simulink model "fs"  (R2021a)
settings: Solver=FixedStepAuto  StartTime=0.0  StopTime=inf  FixedStep=0.05  RelTol=1e-3
undefined symbols (not defined in the file): Angular, Linear
libraries: robotlib x19, simulink x1
settings Model: Creator=ivory  LastModifiedBy=refulgent
settings SolverCC: AlgebraicLoopSolver=TrustRegion
settings OptimizationCC: EnhancedBackFolding=on  PassReuseOutputArgsAs=Individual arguments  ZeroExternalMemoryAtStartup=off  ZeroInternalMemoryAtStartup=off  MaxStackSize=64  OptimizeBlockOrder=speed  DifferentSizesBufferReuse=on  OptimizationCustomize=off  EfficientTunableParamExpr=on
settings DebuggingCC: ParameterTunabilityLossMsg=error  SFMachineParentedDataDiag=warning
settings HardwareCC: ProdBitPerPointer=32  ProdBitPerSizeT=32  ProdBitPerPtrDiffT=32  ProdLargestAtomicFloat=None  ProdIntDivRoundTo=Undefined  ProdEndianess=Unspecified  ProdWordSize=32  ProdHWDeviceType=Generic->Unspecified (assume 32-bit Generic)
settings SFSimCC: MATLABDynamicMemAlloc=off  SimTargetLang=C++
settings RTWCC: SystemTargetFile=ert.tlc  HardwareBoard=Robot Operating System (ROS)  TLCOptions="-aInlineSetEventsForThisBaseRateFcn=TLC_FALSE -aSuppressMultiTaskScheduler=TLC_FALSE  -aRateBasedStepFcn=0"  TemplateMakefile=ert_default_tmf  GenerateReport=on  Toolchain=Catkin  IncludeHyperlinkInReport=on  LaunchReport=on  TargetLang=C++  GenerateTraceInfo=on  GenerateTraceReport=on  GenerateTraceReportSl=on  GenerateTraceReportSf=on  GenerateTraceReportEml=on
settings CodeAppCC: ForceParamTrailComments=on  IgnoreCustomStorageClasses=off  OperatorAnnotations=on  SimulinkDataObjDesc=on  SFDataObjDesc=on  InsertBlockDesc=on
settings ERTTargetCC: SupportContinuousTime=on  SupportVariableSizeSignals=on

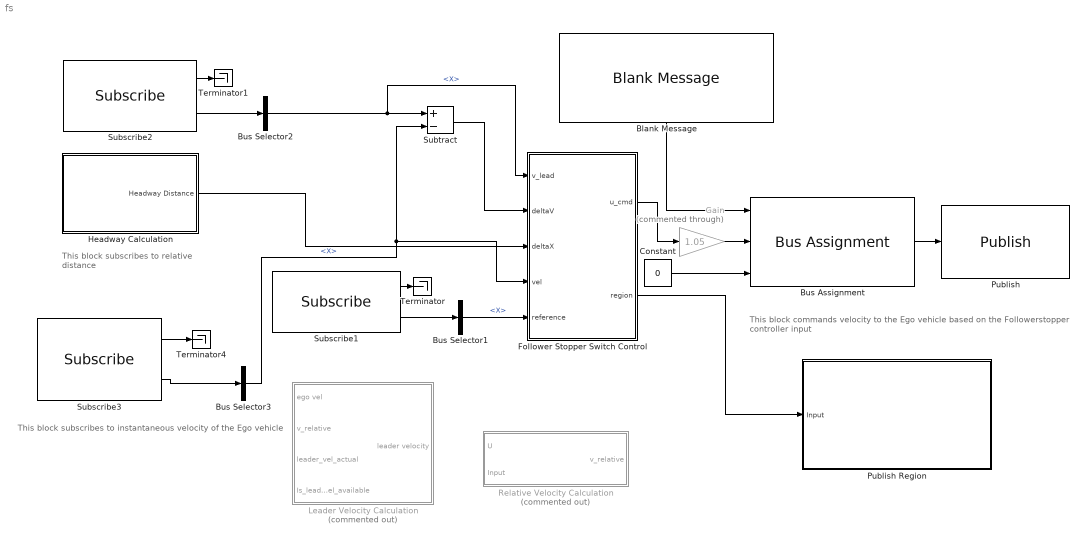
== system fs ==
  note: This block subscribes to
      | instantaneous velocity of the Ego vehicle
  note: This block subscribes
      | to relative distance
  note: This block commands velocity to the Ego vehicle based
      | on the Followerstopper controller input
  Blank Message : robotlib/Blank Message  messageClass=Message  entityType=geometry_msgs/Twist  messageType=geometry_msgs/Twist  SampleTime=inf  legacyBusStruct=off
  Bus Assignment : BusAssignment  AssignedSignals=Linear.X,Angular.Z
  Bus Selector1 : BusSelector  OutputSignals=Linear.X
  Bus Selector2 : BusSelector  OutputSignals=Linear.X
  Bus Selector3 : BusSelector  OutputSignals=Linear.X
  Constant : Constant  Value=0
  Follower Stopper Switch Control : Subsystem
  Gain : Gain  Commented=through  Gain=1.05
  Headway Calculation : Subsystem
  Leader Velocity Calculation : Subsystem  Commented=on
  Publish : robotlib/Publish  topicSource=Specify your own  topic=cmd_vel  messageType=geometry_msgs/Twist  legacyBusStruct=off  messageQueueLength=1
  Publish Region : Subsystem
  Relative Velocity Calculation : Subsystem  Commented=on
  Subscribe1 : robotlib/Subscribe  topicSource=Specify your own  topic=v_ref  messageType=geometry_msgs/Twist  SampleTime=-1  legacyBusStruct=off  messageQueueLength=1
  Subscribe2 : robotlib/Subscribe  topicSource=Specify your own  topic=leader_vel  messageType=geometry_msgs/Twist  SampleTime=-1  legacyBusStruct=off  messageQueueLength=1
  Subscribe3 : robotlib/Subscribe  topicSource=Specify your own  topic=vel  messageType=geometry_msgs/Twist  SampleTime=-1  legacyBusStruct=off  messageQueueLength=1
  Subtract : Sum  Inputs=+-
  Terminator : Terminator
  Terminator1 : Terminator
  Terminator4 : Terminator
  wires:
  Bus Assignment/1 -> Publish/1
  Subscribe3/2 -> Bus Selector3/1
  Blank Message/1 -> Bus Assignment/1
  Bus Selector3/1 -> Subtract/2, Follower Stopper Switch Control/4(vel)  "<X>"
  Constant/1 -> Bus Assignment/3
  Subscribe3/1 -> Terminator4/1
  Follower Stopper Switch Control/1(u_cmd) -> Gain/1
  Gain/1 -> Bus Assignment/2
  Headway Calculation/1(Headway Distance) -> Follower Stopper Switch Control/3(deltaX)
  Bus Selector1/1 -> Follower Stopper Switch Control/5(reference)  "<X>"
  Follower Stopper Switch Control/2(region) -> Publish Region/1(Input)
  Subscribe1/1 -> Terminator/1
  Subscribe1/2 -> Bus Selector1/1
  Subscribe2/2 -> Bus Selector2/1
  Bus Selector2/1 -> Follower Stopper Switch Control/1(v_lead), Subtract/1  "<X>"
  Subtract/1 -> Follower Stopper Switch Control/2(deltaV)
  Subscribe2/1 -> Terminator1/1

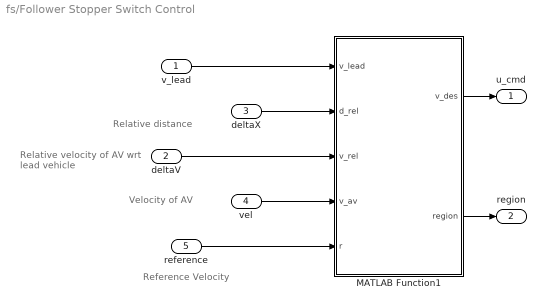
== system fs/Follower Stopper Switch Control ==
  note: Relative velocity of
      | AV wrt lead vehicle
  note: Velocity of AV
  note: Reference Velocity
  note: Relative distance
  v_lead : Inport
  deltaV : Inport  Port=2
  deltaX : Inport  Port=3
  vel : Inport  Port=4
  reference : Inport  Port=5
  MATLAB Function1 : MATLAB Function  TreatAsAtomicUnit=on
  u_cmd : Outport
  region : Outport  Port=2
  wires:
  deltaX/1 -> MATLAB Function1/2(d_rel)
  deltaV/1 -> MATLAB Function1/3(v_rel)
  vel/1 -> MATLAB Function1/4(v_av)
  v_lead/1 -> MATLAB Function1/1(v_lead)
  reference/1 -> MATLAB Function1/5(r)
  MATLAB Function1/1(v_des) -> u_cmd/1
  MATLAB Function1/2(region) -> region/1

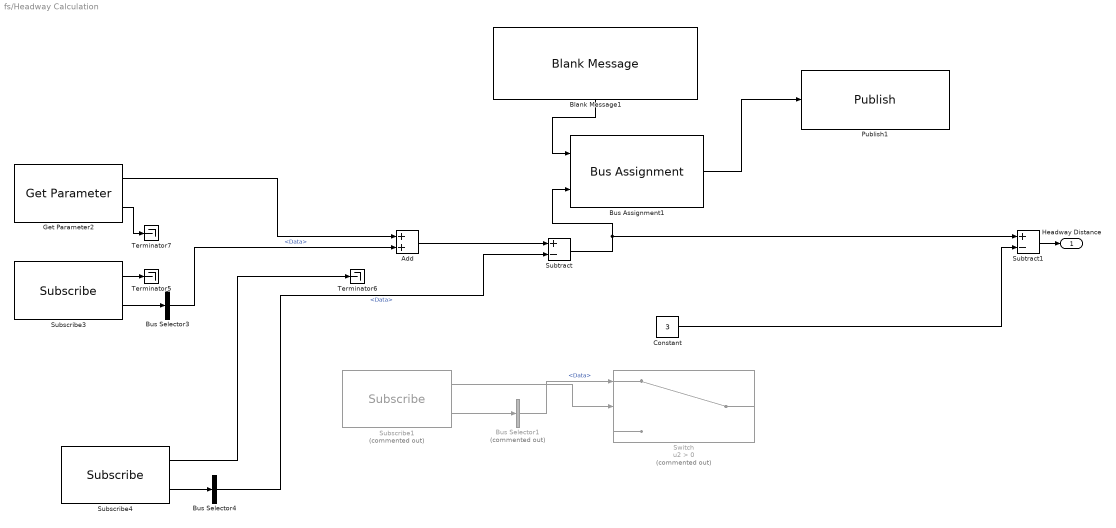
== system fs/Headway Calculation ==
  Add : Sum
  Blank Message1 : robotlib/Blank Message  messageClass=Message  entityType=std_msgs/Float64  messageType=std_msgs/Float64  SampleTime=inf  legacyBusStruct=off
  Bus Assignment1 : BusAssignment  AssignedSignals=Data
  Bus Selector1 : BusSelector  Commented=on  OutputSignals=Data
  Bus Selector3 : BusSelector  OutputSignals=Data
  Bus Selector4 : BusSelector  OutputSignals=Data
  Constant : Constant  Value=3
  Get Parameter2 : robotlib/Get Parameter  ParameterSource=Specify your own  ParameterName=init_gap  ParameterType=double  ParameterMaxArrayLength=16  ParameterInitialValue=30.0  SampleTime=-1  ShowErrorCodeOutput=on  ModelName=fs  BlockId=ParamGet_fs_177
      settings: SourceProductBaseCode=RR
  Publish1 : robotlib/Publish  topicSource=Specify your own  topic=headway_est  messageType=std_msgs/Float64  legacyBusStruct=off  messageQueueLength=1
  Subscribe1 : robotlib/Subscribe  Commented=on  topicSource=Specify your own  topic=headway  messageType=std_msgs/Float64  SampleTime=-1  legacyBusStruct=off  messageQueueLength=1
  Subscribe3 : robotlib/Subscribe  topicSource=Specify your own  topic=leader_dist_x  messageType=std_msgs/Float64  SampleTime=-1  legacyBusStruct=off  messageQueueLength=1
  Subscribe4 : robotlib/Subscribe  topicSource=Specify your own  topic=dist_x  messageType=std_msgs/Float64  SampleTime=-1  legacyBusStruct=off  messageQueueLength=1
  Subtract : Sum  Inputs=+-
  Subtract1 : Sum  Inputs=+-
  Switch : Switch  Commented=on  Criteria=u2 > Threshold
  Terminator5 : Terminator
  Terminator6 : Terminator
  Terminator7 : Terminator
  Headway Distance : Outport
  wires:
  Bus Selector3/1 -> Add/2  "<Data>"
  Subscribe1/2 -> Bus Selector1/1
  Subscribe3/2 -> Bus Selector3/1
  Subscribe4/1 -> Terminator6/1
  Bus Selector1/1 -> Switch/1  "<Data>"
  Subscribe1/1 -> Switch/2
  Bus Selector4/1 -> Subtract/2  "<Data>"
  Get Parameter2/2 -> Terminator7/1
  Subscribe4/2 -> Bus Selector4/1
  Get Parameter2/1 -> Add/1
  Subscribe3/1 -> Terminator5/1
  Add/1 -> Subtract/1
  Subtract/1 -> Subtract1/1, Bus Assignment1/2
  Blank Message1/1 -> Bus Assignment1/1
  Bus Assignment1/1 -> Publish1/1
  Subtract1/1 -> Headway Distance/1
  Constant/1 -> Subtract1/2

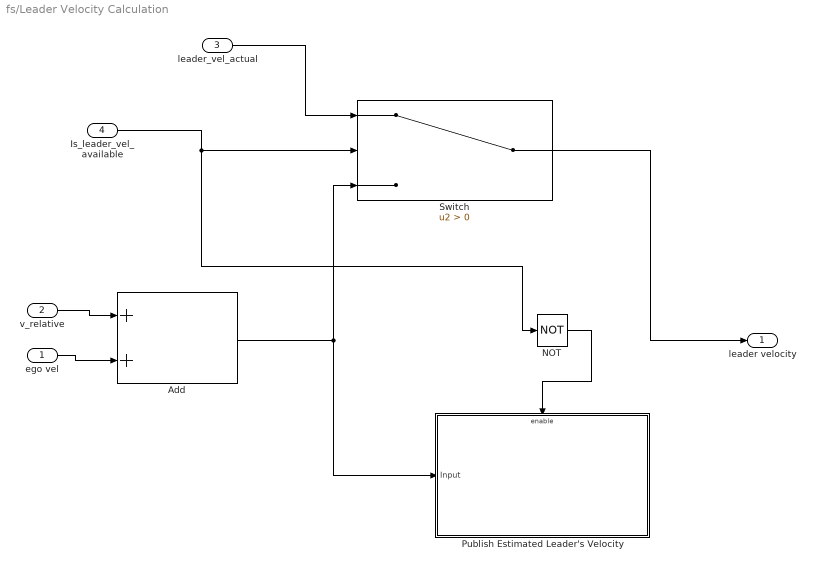
== system fs/Leader Velocity Calculation ==
  ego vel : Inport
  v_relative : Inport  Port=2
  leader_vel_actual : Inport  Port=3
  Is_leader_vel_available : Inport  Port=4
  Add : Sum
  NOT : Logic  Operator=NOT  IconShape=distinctive  AllPortsSameDT=off  OutDataTypeStr=boolean
  Publish Estimated Leader's Velocity : Subsystem
  Switch : Switch  Criteria=u2 > Threshold
  leader velocity : Outport
  wires:
  Add/1 -> Publish Estimated Leader's Velocity/1(Input), Switch/3
  ego vel/1 -> Add/2
  v_relative/1 -> Add/1
  Is_leader_vel_available/1 -> NOT/1, Switch/2
  Switch/1 -> leader velocity/1
  NOT/1 -> Publish Estimated Leader's Velocity/Enable
  leader_vel_actual/1 -> Switch/1

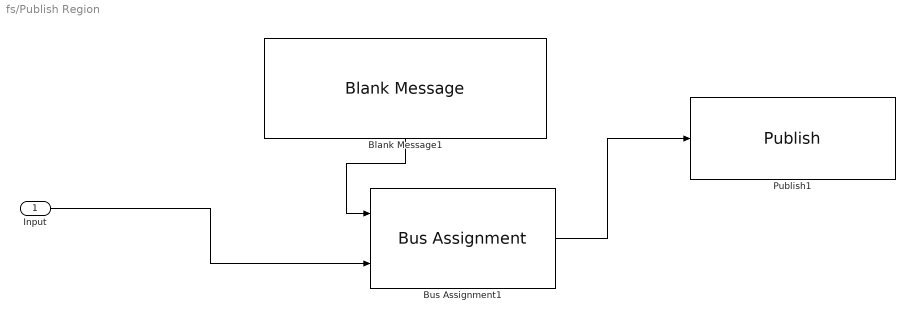
== system fs/Publish Region ==
  Input : Inport
  Blank Message1 : robotlib/Blank Message  messageClass=Message  entityType=std_msgs/UInt8  messageType=std_msgs/UInt8  SampleTime=inf  legacyBusStruct=off
  Bus Assignment1 : BusAssignment  AssignedSignals=Data
  Publish1 : robotlib/Publish  topicSource=Specify your own  topic=region  messageType=std_msgs/UInt8  legacyBusStruct=off  messageQueueLength=1
  wires:
  Input/1 -> Bus Assignment1/2
  Blank Message1/1 -> Bus Assignment1/1
  Bus Assignment1/1 -> Publish1/1

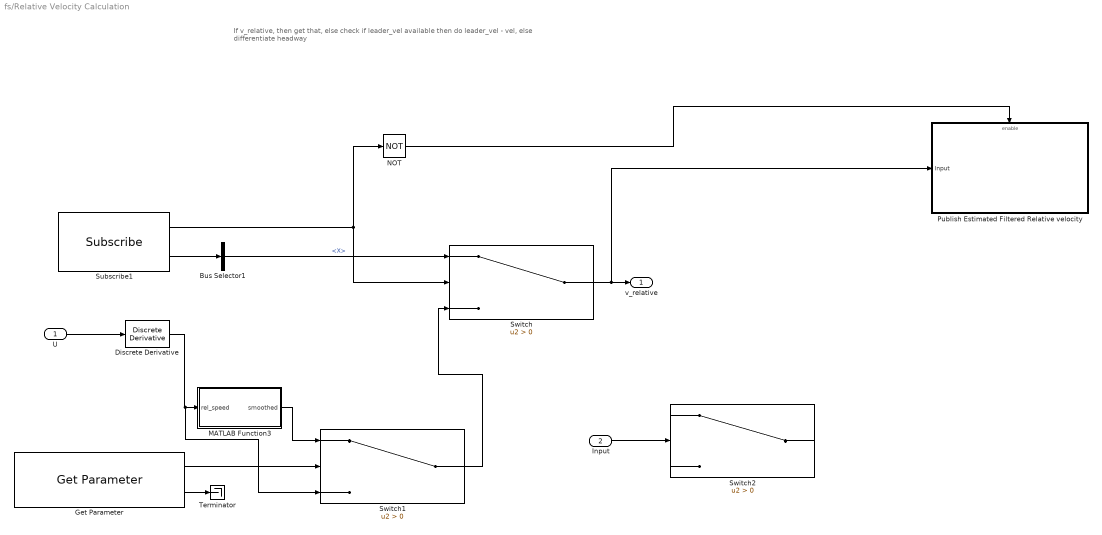
== system fs/Relative Velocity Calculation ==
  note: If v_relative, then get that, else check if leader_vel available then do leader_vel - vel, else differentiate headway
  U : Inport
  Input : Inport  Port=2
  Bus Selector1 : BusSelector  OutputSignals=Linear.X
  Discrete Derivative : simulink/Discrete/Discrete Derivative  gainval=1  ICPrevScaledInput=15.0  OutMin=[]  OutMax=[]  OutDataType=fixdt(1, 16)  OutScaling=2^-10  RndMeth=Convergent  DoSatur=off
  Get Parameter : robotlib/Get Parameter  ParameterSource=Specify your own  ParameterName=HEADWAY_SMOOTHING  ParameterType=boolean  ParameterMaxArrayLength=16  ParameterInitialValue=0.0  SampleTime=-1  ShowErrorCodeOutput=on  ModelName=fs_th  BlockId=ParamGet_fs_th_196
      settings: SourceProductBaseCode=RR
  MATLAB Function3 : MATLAB Function  TreatAsAtomicUnit=on
  NOT : Logic  Operator=NOT  IconShape=distinctive  AllPortsSameDT=off  OutDataTypeStr=boolean
  Publish Estimated Filtered Relative velocity : Subsystem
  Subscribe1 : robotlib/Subscribe  topicSource=Specify your own  topic=v_relative  messageType=geometry_msgs/Twist  SampleTime=-1  legacyBusStruct=off  messageQueueLength=1
  Switch : Switch  Criteria=u2 > Threshold
  Switch1 : Switch  Criteria=u2 > Threshold
  Switch2 : Switch  Criteria=u2 > Threshold
  Terminator : Terminator
  v_relative : Outport
  wires:
  U/1 -> Discrete Derivative/1
  Switch1/1 -> Switch/3
  Discrete Derivative/1 -> Switch1/3, MATLAB Function3/1(rel_speed)
  Subscribe1/2 -> Bus Selector1/1
  Subscribe1/1 -> Switch/2, NOT/1
  Bus Selector1/1 -> Switch/1  "<X>"
  Switch/1 -> Publish Estimated Filtered Relative velocity/1(Input), v_relative/1
  Get Parameter/1 -> Switch1/2
  MATLAB Function3/1(smoothed) -> Switch1/1
  Get Parameter/2 -> Terminator/1
  NOT/1 -> Publish Estimated Filtered Relative velocity/Enable
  Input/1 -> Switch2/2

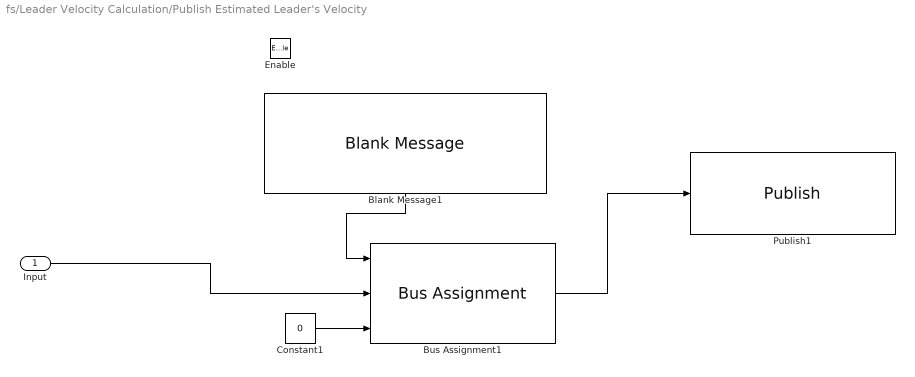
== system fs/Leader Velocity Calculation/Publish Estimated Leader's Velocity ==
  Input : Inport
  Enable : EnablePort
  Blank Message1 : robotlib/Blank Message  messageClass=Message  entityType=geometry_msgs/Twist  messageType=geometry_msgs/Twist  SampleTime=inf  legacyBusStruct=off
  Bus Assignment1 : BusAssignment  AssignedSignals=Linear.X,Angular.Z
  Constant1 : Constant  Value=0
  Publish1 : robotlib/Publish  topicSource=Specify your own  topic=v_leader_est  messageType=geometry_msgs/Twist  legacyBusStruct=off  messageQueueLength=1
  wires:
  Bus Assignment1/1 -> Publish1/1
  Blank Message1/1 -> Bus Assignment1/1
  Constant1/1 -> Bus Assignment1/3
  Input/1 -> Bus Assignment1/2

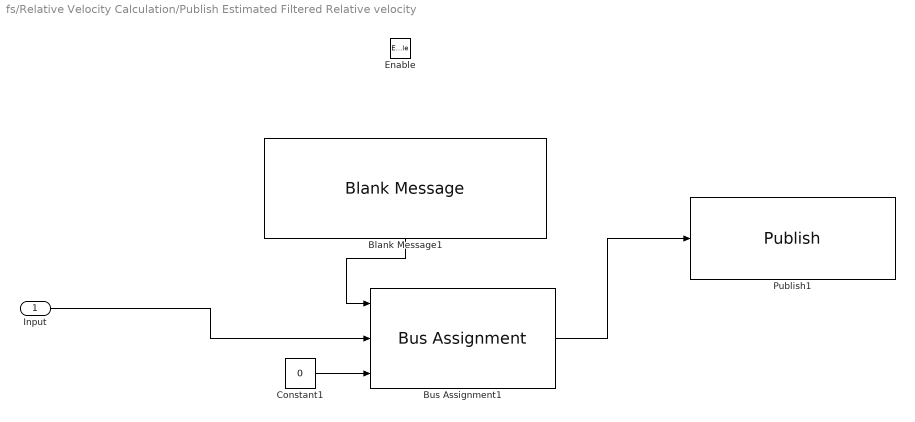
== system fs/Relative Velocity Calculation/Publish Estimated Filtered Relative velocity ==
  Input : Inport
  Enable : EnablePort
  Blank Message1 : robotlib/Blank Message  messageClass=Message  entityType=geometry_msgs/Twist  messageType=geometry_msgs/Twist  SampleTime=inf  legacyBusStruct=off
  Bus Assignment1 : BusAssignment  AssignedSignals=Linear.X,Angular.Z
  Constant1 : Constant  Value=0
  Publish1 : robotlib/Publish  topicSource=Specify your own  topic=v_relative_est  messageType=geometry_msgs/Twist  legacyBusStruct=off  messageQueueLength=1
  wires:
  Input/1 -> Bus Assignment1/2
  Constant1/1 -> Bus Assignment1/3
  Blank Message1/1 -> Bus Assignment1/1
  Bus Assignment1/1 -> Publish1/1

== matlab function fs/Follower Stopper Switch Control/MATLAB Function1 ==
  data: v_lead input; v_des output; d_rel input; v_rel input; v_av input; r input; region output
function [v_des, region]= fcn(v_lead, d_rel,v_rel,v_av, r)
%#codegen
% Safety controller, based on quadratic bands.
% Input: r = desired velocity (from other models)
%          d_rel = estimate of gap to vehicle ahead
%          v_rel = estimate of time derivative of dx (= velocity difference)
%         v_AV = velocity of AV
%      dx_min = minimum distance
% dx_activate = distance below which controller does something
%       decel = vector of three deceleration values for parabolas
% Out:  u_cmd = actual velocity commanded (always u_cmd<=U)
%
% Controller-specific parameters

    w = zeros(3,1);
    alpha = zeros(3,1);
    w(1) = 4.5;
    alpha(1) = 1.5;
    w(3) = 6.0;
    alpha(3) = 0.5;
    w(2) = (w(1)+w(3))/2;
    alpha(2) = (alpha(1)+alpha(3))/2;
    if(nargin<4)
        r = 30;
    end
    
    %v_rel_star = min(v_rel,0)
    v_rel_star = v_rel;
    v_rel_star(v_rel >= 0) = 0;
   
    h_1 = 0.4;
    h_2 = 1.2;
    h_3 = 1.8;
    
    x1 = w(1) + (0.5*v_rel_star.^2)/alpha(1);
    x2 = w(2) + (0.5*v_rel_star.^2)/alpha(2);
    x3 = w(3) + (0.5*v_rel_star.^2)/alpha(3);
    
%     v_lead = v_av+v_rel;
    
    
    %v = min([max([v_lead,0]),r]);
    v = v_lead;
    v(v_lead<0) = 0;
    
    v(v_lead>r) = r;
  
    v_des = zeros(size(d_rel)); 
    %safe region
    v_des(d_rel>x3) = r;  
    %adaptation region 2
    temp_v_des = v+(r-v).*(d_rel-x2)./(x3-x2);
    v_des(d_rel>x2 & d_rel<=x3) = temp_v_des(d_rel>x2 & d_rel<=x3);   
    %adaptation region 1
    temp_v_des = v.*(d_rel-x1)./(x2-x1);
    v_des(d_rel>x1 & d_rel<=x2) = temp_v_des(d_rel>x1 & d_rel<=x2); 
    
    if d_rel>x3
        region = uint8(0);
    elseif d_rel>x2 && d_rel<=x3
        region = uint8(1);
    elseif d_rel>x1 && d_rel<=x2
        region = uint8(2);
    else
        region = uint8(3);
    end

== matlab function fs/Relative Velocity Calculation/MATLAB Function3 ==
  data: rel_speed input; smoothed output
function  smoothed = online_smoothing(rel_speed)

array_length = 75;
window_size = 70;
persistent array

persistent count

if isempty(count)
    count = 0;
else
    
    if count < 75
        count = count + 1;
    end
    
end

if isempty(array)
    array = zeros(1, array_length);
else
    array = [array(2:end), rel_speed];
end

if count < 70
    smoothed = rel_speed;
else
    smoothed_array = smoothdata(array, 'sgolay',window_size);
    smoothed = smoothed_array(end);
end
